simulink subsystem "Pressure_Transducer"  (R2022b)
settings: Solver=VariableStepAuto  StartTime=0.0  StopTime=10.0  RelTol=1e-3
model mask{max_press=5000, lower_val=4, upper_val=20}
  mask prompts: max_press "PT Max Pressure"; lower_val "Upper Signal"; upper_val "Lower Signal"
libraries: fl_lib x2, nesl_utility x1
settings Model: Creator=Owner  LastModifiedBy=Owner

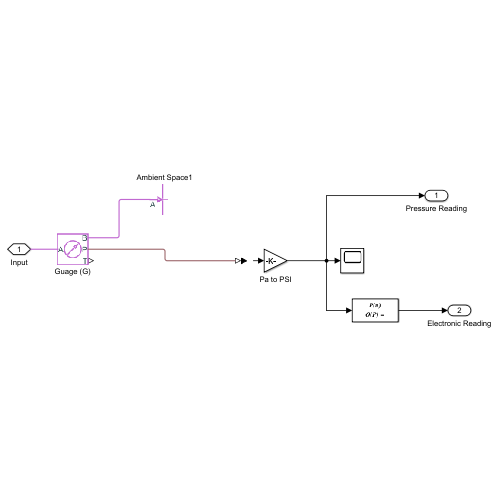
[thumbnail: Simulink's stored preview of the top-level diagram]
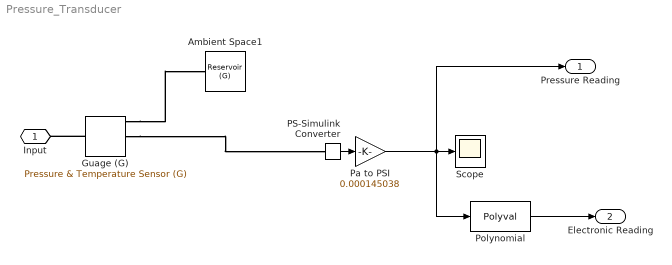
== system Pressure_Transducer ==
  Ambient Space1 : fl_lib/Gas/Elements/Reservoir (G)  pressure_spec=foundation.enum.pressure_spec.atmospheric  reservoir_pressure=0.101325 MPa  reservoir_temperature=293.15 K  area_A=0.01 m^2
  Guage (G) : fl_lib/Gas/Sensors/Pressure & Temperature Sensor (G)
      settings: InternalSimscapePortConfiguration="{\"Bottom\":[],\"Left\":[{\"id\":\"A\",\"label\":\"A\",\"type\":\"foundation.gas.gas\"}],\"Right\":[{\"id\":\"B\",\"label\":\"B\",\"type\":\"foundation.gas.gas\"},{\"id\":\"P\",\"label\":\"P\",\"type\":\"output\"},{\"id\":\"T\",\"label\":\"T\",\"type\":\"output\"}],\"Top\":[]}"
  PS-Simulink Converter : nesl_utility/PS-Simulink Converter  PhysicalDomain=network_engine_domain  SubClassName=ps_output  LeftPortType=input  RightPortType=output  PseudoPeriodic=off  Frequencies=[]  VectorFormat=inherit  Unit=inherit  AffineConversion=off
  Pa to PSI : Gain  Gain=0.000145038
  Polynomial : Polyval  Coefs=[(upper_val-lower_val)/max_press, lower_val]
  Scope : Scope
  Input : PMIOPort  Side=Left
  Pressure Reading : Outport
  Electronic Reading : Outport  Port=2
  wires:
  Polynomial/1 -> Electronic Reading/1
  PS-Simulink Converter/1 -> Pa to PSI/1
  Pa to PSI/1 -> Pressure Reading/1, Polynomial/1, Scope/1
  connections:
  Guage (G)/LConn1 -- Input/RConn1
  Guage (G)/RConn1 -- Ambient Space1/LConn1
  Guage (G)/RConn2 -- PS-Simulink Converter/LConn1
